simulink model "a1__AM_DSB_SC"  (R2019a)
settings: Solver=VariableStepAuto  StartTime=0.0  StopTime=10.0  RelTol=1e-3
libraries: dsparch4 x1
settings Model: Creator=Thanh_Hai  LastModifiedBy=Thanh_Hai

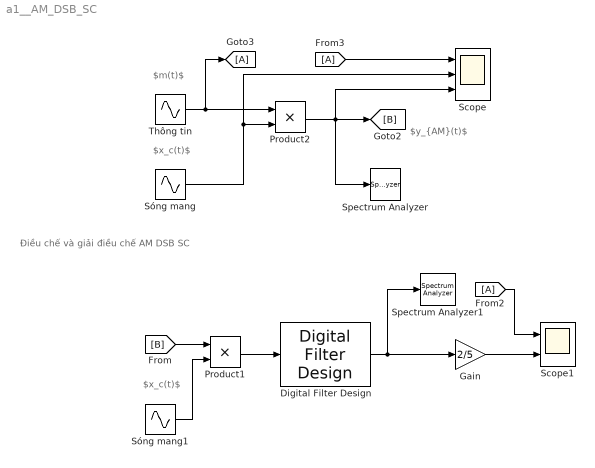
== system a1__AM_DSB_SC ==
  note: $y_{AM}(t)$
  note: $x_c(t)$
  note: $m(t)$
  note: Điều chế và giải điều chế AM DSB SC
  note: $x_c(t)$
  Digital Filter Design : dsparch4/Digital Filter Design  mwdsp_browser_bugfix_var=off
  Gain : Gain  Gain=2/5
  Product1 : Product
  Product2 : Product
  Scope : Scope  NumInputPorts=3
  Scope1 : Scope  NumInputPorts=2
  Spectrum Analyzer : SpectrumAnalyzer
  Spectrum Analyzer1 : SpectrumAnalyzer
  Sóng mang : Sin  Amplitude=5  Frequency=2*pi*5000  SampleTime=1/50000
  Sóng mang1 : Sin  Frequency=2*pi*5000  SampleTime=1/50000
  Thông tin : Sin  Frequency=2*pi*200  SampleTime=1/50000
  wires:
  Sóng mang/1 -> Scope/2, Product2/2
  Thông tin/1 -> Product2/1, [A]
  [A] -> Scope/1
  Product2/1 -> Spectrum Analyzer/1, Scope/3, [B]
  Product1/1 -> Digital Filter Design/1
  Digital Filter Design/1 -> Gain/1, Spectrum Analyzer1/1
  [B] -> Product1/1
  Sóng mang1/1 -> Product1/2
  [A] -> Scope1/1
  Gain/1 -> Scope1/2
